simulink model "BR_Test_Star"  (R2020a)
settings: Solver=VariableStepAuto  StartTime=0.0  StopTime=2  RelTol=1e-3
libraries: powerlib x11, powerlib_meascontrol x3
settings Model: Creator=krishna  LastModifiedBy=krishna

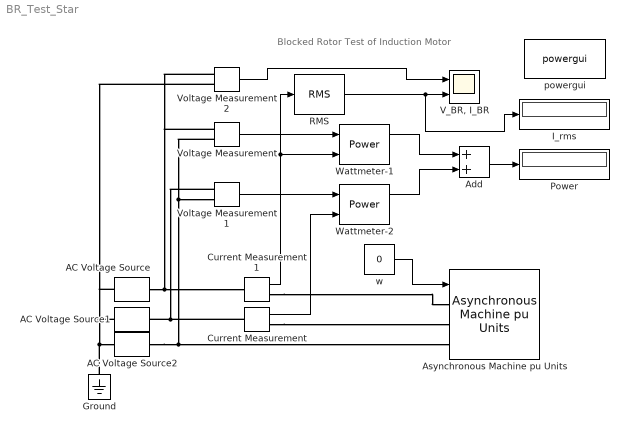
== system BR_Test_Star ==
  note: Blocked Rotor Test of Induction Motor
  AC Voltage Source : powerlib/Electrical Sources/AC Voltage Source  Amplitude=39.5  Phase=0  Frequency=50  SampleTime=0  Measurements=None  BusType=swing  Pref=10e3  Qref=0  Qmin=-inf  Qmax=+inf
  AC Voltage Source1 : powerlib/Electrical Sources/AC Voltage Source  Amplitude=39.5  Phase=120  Frequency=50  SampleTime=0  Measurements=None  BusType=swing  Pref=10e3  Qref=0  Qmin=-inf  Qmax=+inf
  AC Voltage Source2 : powerlib/Electrical Sources/AC Voltage Source  Amplitude=39.5  Phase=-120  Frequency=50  SampleTime=0  Measurements=None  BusType=swing  Pref=10e3  Qref=0  Qmin=-inf  Qmax=+inf
  Add : Sum
  Asynchronous Machine pu Units : powerlib/Machines/Asynchronous Machine pu Units  RotorType=Squirrel-cage  PresetModel=No  MechanicalLoad=Speed w  ShowDetailedParameters=on  ReferenceFrame=Rotor  Units=pu  MeasurementBus=on  NominalParameters=[7460 415 50]  Stator=[0.01965 0.0397]  Rotor=[0.01909 0.0397]  Cage1=[0.01909 0.0397]  Cage2=[0.01909 0.0397]  Lm=1.354  Mechanical=[0.09526 0.05479 2]  PolePairs=2  InitialConditions="[ 1,0   0,0,0   0,0,0 ]"  SimulateSaturation=off  Saturation="[0.212,0.4201,0.8125,1.0979,1.4799,2.2457,3.2586,4.5763,6.4763 ;   0.5,0.7,0.9,1,1.1,1.2 ,1.3,1.4,1.5]"  LoadFlowParameters=0  TsPowergui=0  TsBlock=-1  IterativeModel=Trapezoidal non iterative  IterativeDiscreteModel=Trapezoidal non iterative  Pmec=0
      settings: SourceProductBaseCode=PS
  Current Measurement : powerlib/Measurements/Current Measurement  PhasorSimulation=off  OutputType=Complex  PSBequivalent=0
  Current Measurement1 : powerlib/Measurements/Current Measurement  PhasorSimulation=off  OutputType=Complex  PSBequivalent=0
  Ground : powerlib/Elements/Ground  LConnTagsString=a
  I_rms : Display
  Power : Display
  RMS : powerlib_meascontrol/Measurements/RMS  TrueRMS=on  Freq=50  RMSInit=0  Ts=0
  "V_BR, I_BR" : Scope  NumInputPorts=2
  Voltage Measurement : powerlib/Measurements/Voltage Measurement  PhasorSimulation=off  OutputType=Complex  PSBequivalent=0
  Voltage Measurement1 : powerlib/Measurements/Voltage Measurement  PhasorSimulation=off  OutputType=Complex  PSBequivalent=0
  Voltage Measurement2 : powerlib/Measurements/Voltage Measurement  PhasorSimulation=off  OutputType=Complex  PSBequivalent=0
  Wattmeter-1 : powerlib_meascontrol/Measurements/Power  Freq=50  Vinit=[1, 0]  Iinit=[1, 0]  Ts=0
  Wattmeter-2 : powerlib_meascontrol/Measurements/Power  Freq=50  Vinit=[1, 0]  Iinit=[1, 0]  Ts=0
  powergui : powerlib/powergui  Priority=1  SimulationMode=Continuous  SampleTime=50e-6  frequency=60  Iterations=50  frequencyindice=50  Pbase=100e6  ErrMax=1e-4  UnitsV=kV  UnitsW=MW  buscounter=0  FunctionMessages=off  echomessages=off  EnableUseOfTLC=off  CurrentSourceSwitches=off  DisableSnubberDevices=off  DisableRonSwitches=off  DisableVfSwitches=off  DisplayEquations=off  AutomaticDiscreteSolvers=off  SolverType=Tustin/Backward Euler (TBE)  Interpol=off  ExternalGateDelay=off  methode=off  Ts=100  x0status=blocks  SPID=on  SwTol=0  HookPort=off  NonlinearTolerance=1e-4  nMaxIteration=100  ContinueOnMaxIteration=off  RestoreLinks=warning  ResistiveCurrentMeasurement=off  Frange=[0:2:500]  Ylog=off  Xlog=on  ShowGrid=off  save=off  variable=ZData  structure=0  ZoomFFT=off  StartTime=0.0  cycles=1  DisplayStyle=1  fundamental=60  FreqAxis=off  MaxFrequency=1000  frequencyindicesteady=1  RmsSteady=1  display=off
  w : Constant  Value=0
  wires:
  Voltage Measurement/1 -> Wattmeter-1/1
  Current Measurement1/1 -> RMS/1, Wattmeter-1/2
  Voltage Measurement1/1 -> Wattmeter-2/1
  Current Measurement/1 -> Wattmeter-2/2
  Wattmeter-1/1 -> Add/1
  Wattmeter-2/1 -> Add/2
  Add/1 -> Power/1
  w/1 -> Asynchronous Machine pu Units/1
  RMS/1 -> I_rms/1, "V_BR, I_BR"/2
  Voltage Measurement2/1 -> "V_BR, I_BR"/1
  connections:
  Voltage Measurement/LConn2 -- AC Voltage Source2/RConn1 -- Asynchronous Machine pu Units/LConn3 -- Voltage Measurement1/LConn2
  Voltage Measurement2/LConn2 -- AC Voltage Source/LConn1 -- AC Voltage Source1/LConn1 -- Ground/LConn1 -- AC Voltage Source2/LConn1
  Current Measurement/RConn1 -- Asynchronous Machine pu Units/LConn2
  Current Measurement/LConn1 -- Voltage Measurement1/LConn1 -- AC Voltage Source1/RConn1
  Current Measurement1/RConn1 -- Asynchronous Machine pu Units/LConn1
  AC Voltage Source/RConn1 -- Voltage Measurement2/LConn1 -- Voltage Measurement/LConn1 -- Current Measurement1/LConn1
